simulink model "lineal_model"  (R2015a)
settings: Solver=ode45  StartTime=0.0  StopTime=0.1  RelTol=1e-3
values from neighbouring files (symbols this model uses):
  A = A1    [Final_2.m]    (also in Final_discreto.m)
  Ao = Aaum-L*Caum    [Final_2.m]
  B = B1    [Final_2.m]    (also in Final_discreto.m)
  Bo = [Baum L]    [Final_2.m]
  Co = [eye(size(Ao,1)-1) zeros(size(Ao,1)-1,1)]    [Final_2.m]
  Do = zeros(size(Ao,1)-1,2)    [Final_2.m]
  ki = Ki_(5,1)    [Final_2.m]
  ks = [Ki_(1,1) Ki_(2,1) Ki_(3,1) Ki_(4,1) ]'    [Final_2.m]
settings Model: Creator=berme_000  LastModifiedBy=berme_000

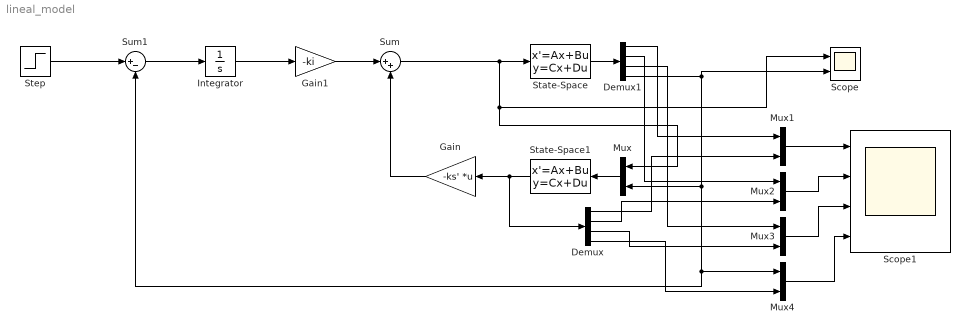
== system lineal_model ==
  Demux : Demux
  Demux1 : Demux
  Gain : Gain  Gain=-ks'  Multiplication=Matrix(K*u)
  Gain1 : Gain  Gain=-ki
  Integrator : Integrator
  Mux{,1..4} (5 alike) : Mux  Inputs=2
  Scope : Scope  NumInputPorts=2
      settings: YMin=-0.5~-5  YMax=10~5  SaveName=lqg_lm_output
  Scope1 : Scope  NumInputPorts=4
      settings: YMin=-8.13152e-20~-0.00075~-5~-5  YMax=0.0015~0.00075~5~5
  State-Space : StateSpace  A=A  B=B  C=eye(4)  D=zeros(4,1)  X0=[.1 -.01 .2 -.1]
  State-Space1 : StateSpace  A=Ao  B=Bo  C=Co  D=Do  X0=0
  Step : Step  Time=0.05  Before=20  After=25  SampleTime=0
  Sum : Sum  Inputs=|++
  Sum1 : Sum  Inputs=|+-
  wires:
  Demux1/4 -> Scope/2, Mux/2, Mux4/1, Sum1/2
  Mux/1 -> State-Space1/1
  Sum/1 -> Scope/1, Mux/1, State-Space/1
  State-Space1/1 -> Demux/1, Gain/1
  Integrator/1 -> Gain1/1
  Gain1/1 -> Sum/1
  Gain/1 -> Sum/2
  Sum1/1 -> Integrator/1
  Step/1 -> Sum1/1
  State-Space/1 -> Demux1/1
  Mux1/1 -> Scope1/1
  Mux2/1 -> Scope1/2
  Mux3/1 -> Scope1/3
  Mux4/1 -> Scope1/4
  Demux1/1 -> Mux1/1
  Demux/1 -> Mux1/2
  Demux1/2 -> Mux2/1
  Demux1/3 -> Mux3/1
  Demux/2 -> Mux2/2
  Demux/3 -> Mux3/2
  Demux/4 -> Mux4/2
